simulink model "P_dual"  (R2021a)
settings: Solver=FixedStepAuto  StartTime=0.0  StopTime=Inf  FixedStep=0.01  RelTol=1e-3  EnableMultiTasking=on
undefined symbols (not defined in the file): DiscIntNeverNeededParam
libraries: arduinolib x10, simulink x2
settings Model: SILPILModeSetting=veronly  ExtModeTrigDuration=2  Creator=Simón  LastModifiedBy=Simón
settings OptimizationCC: EnhancedBackFolding=on  PassReuseOutputArgsAs=Individual arguments  ZeroExternalMemoryAtStartup=off  ZeroInternalMemoryAtStartup=off  MaxStackSize=64  OptimizeBlockOrder=speed  DifferentSizesBufferReuse=on  OptimizationCustomize=off  EfficientTunableParamExpr=on
settings DebuggingCC: ParameterTunabilityLossMsg=error
settings HardwareCC: ProdBitPerInt=16  ProdBitPerPointer=16  ProdBitPerSizeT=16  ProdBitPerPtrDiffT=16  ProdLargestAtomicFloat=None  ProdWordSize=8  ProdHWDeviceType=Atmel->AVR  UseEmbeddedCoderFeatures=off  UseSimulinkCoderFeatures=off
settings SFSimCC: MATLABDynamicMemAlloc=off
settings RTWCC: SystemTargetFile=ert.tlc  HardwareBoard=Arduino Uno  TemplateMakefile=ert_default_tmf  Toolchain=Arduino AVR  BuildConfiguration=Faster Runs
settings CodeAppCC: ForceParamTrailComments=on  IgnoreCustomStorageClasses=off  OperatorAnnotations=on  SimulinkDataObjDesc=on  SFDataObjDesc=on  InsertBlockDesc=on
settings ERTTargetCC: SupportContinuousTime=on  SupportNonInlinedSFcns=on  SupportVariableSizeSignals=on  ExtModeStaticAllocSize=250

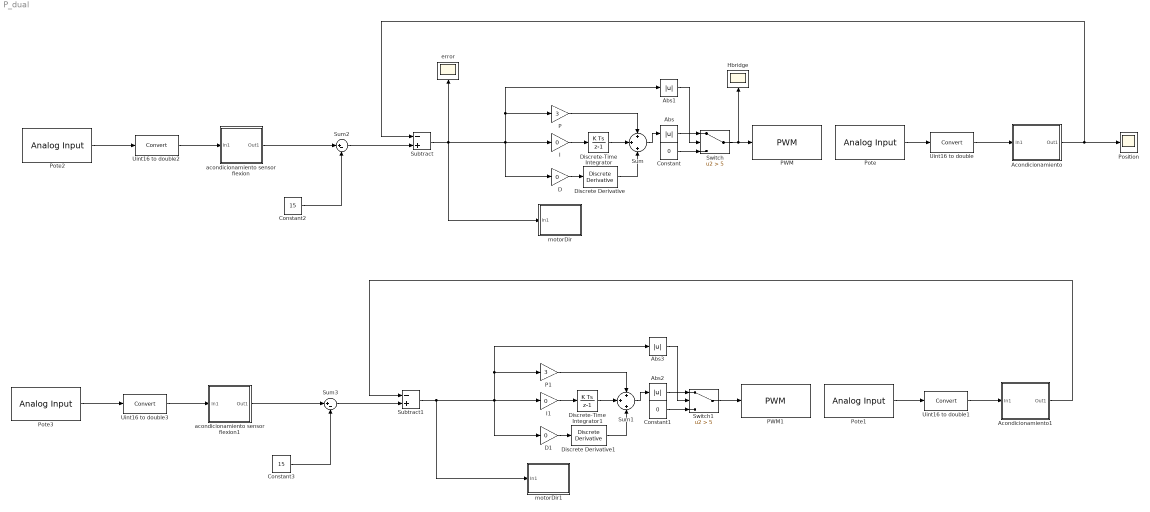
== system P_dual ==
  Abs{,1..3} (4 alike) : Abs
  Acondicionamiento : Subsystem
  Acondicionamiento1 : Subsystem
  Constant : Constant  Value=0
  Constant1 : Constant  Value=0
  Constant2 : Constant  Value=15
  Constant3 : Constant  Value=15
  D : Gain  Gain=0
  D1 : Gain  Gain=0
  Discrete Derivative : simulink/Discrete/Discrete Derivative  gainval=1.0  ICPrevScaledInput=0.0  OutMin=[]  OutMax=[]  OutDataType=fixdt(1, 16)  OutScaling=2^-10  DoSatur=off
  Discrete Derivative1 : simulink/Discrete/Discrete Derivative  gainval=1.0  ICPrevScaledInput=0.0  OutMin=[]  OutMax=[]  OutDataType=fixdt(1, 16)  OutScaling=2^-10  DoSatur=off
  Discrete-Time Integrator : DiscreteIntegrator  SampleTime=-1  ICPrevOutput=DiscIntNeverNeededParam  ICPrevScaledInput=DiscIntNeverNeededParam
  Discrete-Time Integrator1 : DiscreteIntegrator  SampleTime=-1  ICPrevOutput=DiscIntNeverNeededParam  ICPrevScaledInput=DiscIntNeverNeededParam
  Hbridge : Scope
  I : Gain  Gain=0
  I1 : Gain  Gain=0
  P : Gain  Gain=3
  P1 : Gain  Gain=3
  PWM : arduinolib/PWM  pinNumber=10  frequencyType=Default  desiredFrequency=490.2  achievableFrequency=490.2
  PWM1 : arduinolib/PWM  pinNumber=3  frequencyType=Default  desiredFrequency=490.2  achievableFrequency=490.2
  Position : Scope
  Pote : arduinolib/Analog Input  pinNumber=0  ReadResultsOnly=off  ConversionTriggerSource=Software  ExternalTriggerType=uint32( 0 )  OutputDataType=uint16  EnableConversionCompleteNotify=off  EnableOuputStatus=off  SampleTime=-1  blockPlatform=arduino
  Pote1 : arduinolib/Analog Input  pinNumber=3  ReadResultsOnly=off  ConversionTriggerSource=Software  ExternalTriggerType=uint32( 0 )  OutputDataType=uint16  EnableConversionCompleteNotify=off  EnableOuputStatus=off  SampleTime=-1  blockPlatform=arduino
  Pote2 : arduinolib/Analog Input  pinNumber=1  ReadResultsOnly=off  ConversionTriggerSource=Software  ExternalTriggerType=uint32( 0 )  OutputDataType=uint16  EnableConversionCompleteNotify=off  EnableOuputStatus=off  SampleTime=-1  blockPlatform=arduino
  Pote3 : arduinolib/Analog Input  pinNumber=4  ReadResultsOnly=off  ConversionTriggerSource=Software  ExternalTriggerType=uint32( 0 )  OutputDataType=uint16  EnableConversionCompleteNotify=off  EnableOuputStatus=off  SampleTime=-1  blockPlatform=arduino
  Subtract : Sum  Inputs=-+
  Subtract1 : Sum  Inputs=-+
  Sum : Sum  Inputs=+|+|+
  Sum1 : Sum  Inputs=+|+|+
  Sum2 : Sum  Inputs=|+-
  Sum3 : Sum  Inputs=|+-
  Switch : Switch  Criteria=u2 > Threshold  Threshold=5
  Switch1 : Switch  Criteria=u2 > Threshold  Threshold=5
  Uint16 to double{,1..3} (4 alike) : DataTypeConversion
  acondicionamiento sensor flexion : Subsystem
  acondicionamiento sensor flexion1 : Subsystem
  error : Scope
  motorDir : Subsystem
  motorDir1 : Subsystem
  wires:
  Pote/1 -> Uint16 to double/1
  Uint16 to double/1 -> Acondicionamiento/1(In1)
  Sum2/1 -> Subtract/2
  Sum/1 -> Abs/1
  Discrete-Time Integrator/1 -> Sum/2
  I/1 -> Discrete-Time Integrator/1
  P/1 -> Sum/1
  Acondicionamiento/1(Out1) -> Subtract/1, Position/1
  Constant/1 -> Switch/3
  Abs1/1 -> Switch/2
  Subtract/1 -> D/1, Abs1/1, P/1, I/1, motorDir/1(In1), error/1
  Abs/1 -> Switch/1
  Switch/1 -> Hbridge/1, PWM/1
  D/1 -> Discrete Derivative/1
  Discrete Derivative/1 -> Sum/3
  Switch1/1 -> PWM1/1
  D1/1 -> Discrete Derivative1/1
  Discrete Derivative1/1 -> Sum1/3
  Abs2/1 -> Switch1/1
  Abs3/1 -> Switch1/2
  Constant1/1 -> Switch1/3
  P1/1 -> Sum1/1
  Uint16 to double1/1 -> Acondicionamiento1/1(In1)
  Acondicionamiento1/1(Out1) -> Subtract1/1
  Sum3/1 -> Subtract1/2
  Discrete-Time Integrator1/1 -> Sum1/2
  Pote1/1 -> Uint16 to double1/1
  Subtract1/1 -> D1/1, Abs3/1, P1/1, I1/1, motorDir1/1(In1)
  Sum1/1 -> Abs2/1
  I1/1 -> Discrete-Time Integrator1/1
  Uint16 to double2/1 -> acondicionamiento sensor flexion/1(In1)
  acondicionamiento sensor flexion/1(Out1) -> Sum2/1
  Constant2/1 -> Sum2/2
  Pote2/1 -> Uint16 to double2/1
  Uint16 to double3/1 -> acondicionamiento sensor flexion1/1(In1)
  acondicionamiento sensor flexion1/1(Out1) -> Sum3/1
  Constant3/1 -> Sum3/2
  Pote3/1 -> Uint16 to double3/1

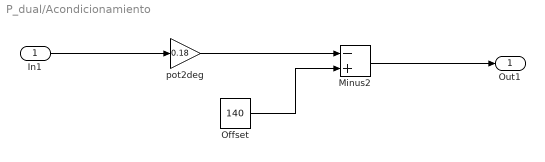
== system P_dual/Acondicionamiento ==
  In1 : Inport
  Minus2 : Sum  Inputs=-+
  Offset : Constant  Value=140
  pot2deg : Gain  Gain=0.18
  Out1 : Outport
  wires:
  Offset/1 -> Minus2/2
  pot2deg/1 -> Minus2/1
  Minus2/1 -> Out1/1
  In1/1 -> pot2deg/1

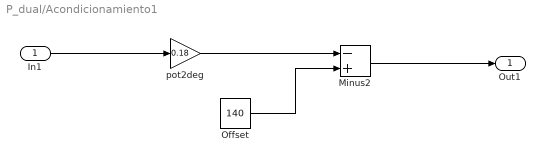
== system P_dual/Acondicionamiento1 ==
  In1 : Inport
  Minus2 : Sum  Inputs=-+
  Offset : Constant  Value=140
  pot2deg : Gain  Gain=0.18
  Out1 : Outport
  wires:
  Offset/1 -> Minus2/2
  pot2deg/1 -> Minus2/1
  Minus2/1 -> Out1/1
  In1/1 -> pot2deg/1

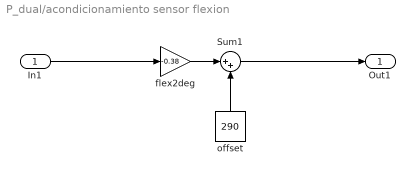
== system P_dual/acondicionamiento sensor flexion ==
  In1 : Inport
  Sum1 : Sum  Inputs=|++
  flex2deg : Gain  Gain=-0.38
  offset : Constant  Value=290
  Out1 : Outport
  wires:
  In1/1 -> flex2deg/1
  offset/1 -> Sum1/2
  flex2deg/1 -> Sum1/1
  Sum1/1 -> Out1/1

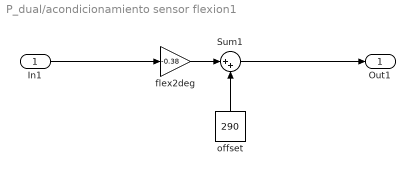
== system P_dual/acondicionamiento sensor flexion1 ==
  In1 : Inport
  Sum1 : Sum  Inputs=|++
  flex2deg : Gain  Gain=-0.38
  offset : Constant  Value=290
  Out1 : Outport
  wires:
  In1/1 -> flex2deg/1
  offset/1 -> Sum1/2
  flex2deg/1 -> Sum1/1
  Sum1/1 -> Out1/1

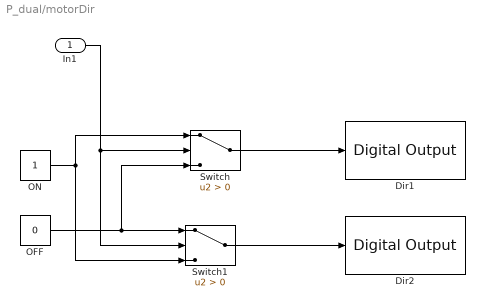
== system P_dual/motorDir ==
  In1 : Inport
  Dir1 : arduinolib/Digital Output  pinNumber=8  Direction=output  blockPlatform=arduino
  Dir2 : arduinolib/Digital Output  pinNumber=9  Direction=output  blockPlatform=arduino
  OFF : Constant  Value=0
  ON : Constant
  Switch : Switch  Criteria=u2 > Threshold
  Switch1 : Switch  Criteria=u2 > Threshold
  wires:
  In1/1 -> Switch1/2, Switch/2
  OFF/1 -> Switch/3, Switch1/1
  ON/1 -> Switch1/3, Switch/1
  Switch1/1 -> Dir2/1
  Switch/1 -> Dir1/1

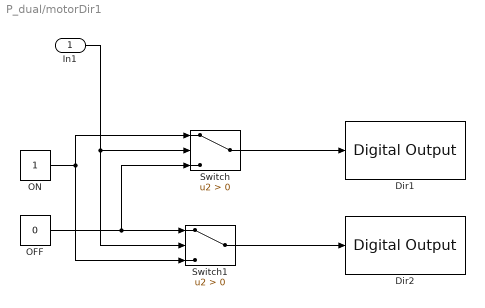
== system P_dual/motorDir1 ==
  In1 : Inport
  Dir1 : arduinolib/Digital Output  pinNumber=6  Direction=output  blockPlatform=arduino
  Dir2 : arduinolib/Digital Output  pinNumber=7  Direction=output  blockPlatform=arduino
  OFF : Constant  Value=0
  ON : Constant
  Switch : Switch  Criteria=u2 > Threshold
  Switch1 : Switch  Criteria=u2 > Threshold
  wires:
  In1/1 -> Switch1/2, Switch/2
  OFF/1 -> Switch/3, Switch1/1
  ON/1 -> Switch1/3, Switch/1
  Switch1/1 -> Dir2/1
  Switch/1 -> Dir1/1
